simulink model "Planar_Full_System_NL"  (R2016a)
settings: Solver=FixedStepAuto  SolverMode=SingleTasking  StartTime=0.0  StopTime=20  RelTol=1e-3
values from neighbouring files (symbols this model uses):
  T_x_AP = 0    [Computation_Reduced_Model.m]    (also in Untitled.m)
  T_y_AP = 0    [Computation_Reduced_Model.m]    (also in Untitled.m)
  T_z_AP = 0    [Computation_Reduced_Model.m]    (also in Untitled.m)
  x_AP = [0;0;0]    [Computation_Reduced_Model.m]    (also in One_ZRM.m = [0;0;0;0;0;0]; Untitled.m)
undefined symbols (not defined in the file or in its folder): K_xz, K_yz
settings Model: Creator=Florian  LastModifiedBy=Florian
settings OptimizationCC: DefaultParameterBehavior=Inlined  UseDivisionForNetSlopeComputation=on  UseFloatMulNetSlope=on  InlineInvariantSignals=on  PassReuseOutputArgsAs=Individual arguments  ZeroExternalMemoryAtStartup=off  ZeroInternalMemoryAtStartup=off  NoFixptDivByZeroProtection=on  EfficientFloat2IntCast=on  OptimizeModelRefInitCode=on  LifeSpan=1
settings HardwareCC: ProdBitPerPointer=32  ProdLargestAtomicInteger=Long  ProdLargestAtomicFloat=Double  ProdWordSize=32  ProdHWDeviceType=ARM Compatible->ARM Cortex
settings RTWCC: SystemTargetFile=ert.tlc  TemplateMakefile=ert_default_tmf  GenerateReport=on  IncludeHyperlinkInReport=on  LaunchReport=on  GenerateTraceInfo=on  GenerateTraceReport=on  GenerateTraceReportSl=on  GenerateTraceReportSf=on  GenerateTraceReportEml=on  GenerateCodeMetricsReport=on
settings CodeAppCC: ForceParamTrailComments=on  IgnoreCustomStorageClasses=off  OperatorAnnotations=on  SimulinkDataObjDesc=on  SFDataObjDesc=on  MATLABFcnDesc=on  InsertBlockDesc=on  MATLABSourceComments=on
settings ERTTargetCC: GenerateSampleERTMain=on  IncludeMdlTerminateFcn=off  CombineSignalStateStructs=on  SupportComplex=off  SupportContinuousTime=on  InlinedParameterPlacement=NonHierarchical  ERTCustomFileTemplate=example_file_process.tlc  ERTFilePackagingFormat=CompactWithDataFile

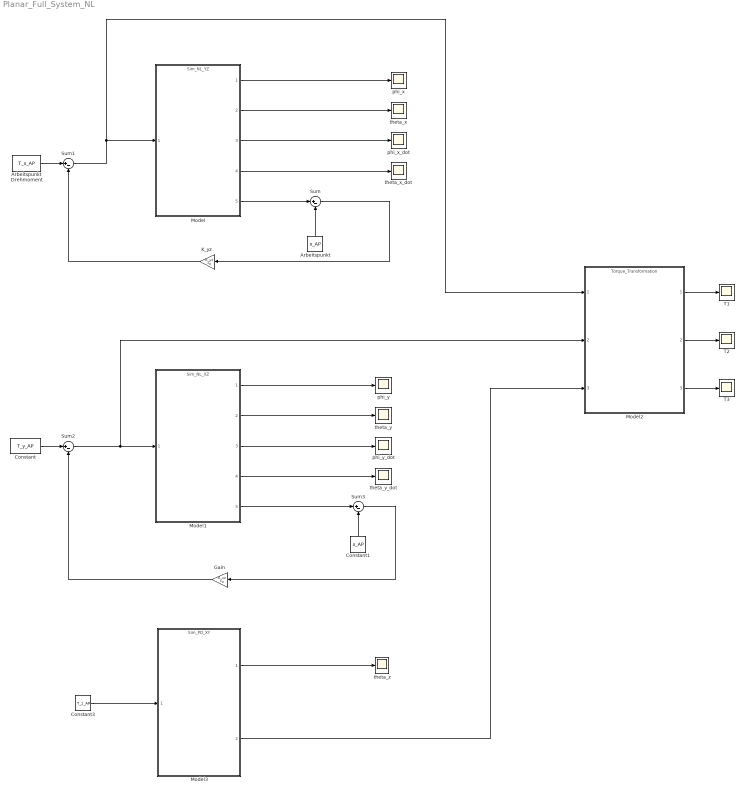
== system Planar_Full_System_NL ==
  Arbeitspunkt : Constant  Value=x_AP
  Arbeitspunkt Drehmoment : Constant  Value=T_x_AP
  Constant : Constant  Value=T_y_AP
  Constant1 : Constant  Value=x_AP
  Constant3 : Constant  Value=T_z_AP
  Gain : Gain  Gain=K_xz  Multiplication=Matrix(K*u) (u vector)
  K_yz : Gain  Gain=K_yz  Multiplication=Matrix(K*u) (u vector)
  Model : ModelReference  ModelNameDialog=Sim_NL_YZ.slx  SimulationMode=Normal  ModelReferenceVersion=1.30
  Model1 : ModelReference  ModelNameDialog=Sim_NL_XZ.slx  SimulationMode=Normal  ModelReferenceVersion=1.11
  Model2 : ModelReference  ModelNameDialog=Torque_Transformation.slx  SimulationMode=Normal  ModelReferenceVersion=1.6
  Model3 : ModelReference  ModelNameDialog=Sim_PD_XY.slx  SimulationMode=Normal  ModelReferenceVersion=1.12
  Sum{,1..3} (4 alike) : Sum  Inputs=|+-
  T1 : Scope
  T2 : Scope
  T3 : Scope
  phi_x : Scope
  phi_x_dot : Scope
  phi_y : Scope
  phi_y_dot : Scope
  theta_x : Scope
  theta_x_dot : Scope
  theta_y : Scope
  theta_y_dot : Scope
  "theta_z " : Scope
  wires:
  Model/1 -> phi_x/1
  Model/2 -> theta_x/1
  Model/3 -> phi_x_dot/1
  Model/4 -> theta_x_dot/1
  Model/5 -> Sum/1
  K_yz/1 -> Sum1/2
  Arbeitspunkt Drehmoment/1 -> Sum1/1
  Arbeitspunkt/1 -> Sum/2
  Sum/1 -> K_yz/1
  Model1/1 -> phi_y/1
  Model1/2 -> theta_y/1
  Model1/3 -> phi_y_dot/1
  Model1/4 -> theta_y_dot/1
  Model1/5 -> Sum3/1
  Constant1/1 -> Sum3/2
  Constant/1 -> Sum2/1
  Gain/1 -> Sum2/2
  Sum2/1 -> Model2/2, Model1/1
  Sum1/1 -> Model2/1, Model/1
  Model2/1 -> T1/1
  Model2/2 -> T2/1
  Model2/3 -> T3/1
  Constant3/1 -> Model3/1
  Model3/1 -> "theta_z "/1
  Model3/2 -> Model2/3
  Sum3/1 -> Gain/1
